simulink model "stepinsim"  (R2018b)
settings: Solver=VariableStepAuto  StartTime=0.0  StopTime=10.0  RelTol=1e-3
libraries: fuzblock x1
settings Model: Creator=student  LastModifiedBy=student

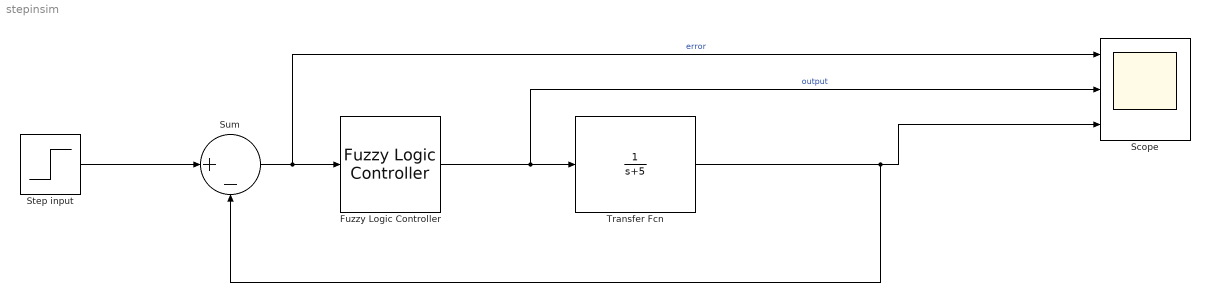
== system stepinsim ==
  Fuzzy Logic Controller : fuzblock/Fuzzy Logic  Controller  FIS=stepin  OutputSampleNumber=101  DataType=double  FuzzifiedInputs=off  RuleFiringStrengths=off  RuleOutputs=off  AggregatedOutputs=off  SimulateUsing=Interpreted execution  OutOfRangeInputValueMessage=warning  NoRuleFiredMessage=warning  EmptyOutputFuzzySetMessage=warning
  Scope : Scope  NumInputPorts=3
  Step input : Step  SampleTime=0
  Sum : Sum  Inputs=|+-
  Transfer Fcn : TransferFcn  Denominator=[1 5]
  wires:
  Step input/1 -> Sum/1
  Fuzzy Logic Controller/1 -> Scope/2, Transfer Fcn/1  "output"
  Sum/1 -> Scope/1, Fuzzy Logic Controller/1  "error"
  Transfer Fcn/1 -> Sum/2, Scope/3
